simulink library "PowerFlowLib"  (R2016a)
settings: Solver=ode45  StartTime=0.0  StopTime=10.0  RelTol=1e-3
undefined symbols (not defined in the file or in its folder): Air, AirProp, C, F1, F2, Fanmap, Fld1, Fld2, Fluid, fueltankdata, HydProp, HydraulicLoad, IBFD_exc, L, LoadFluidProps, magnitude, MSSN, n_alghts, PumpProp, pwr_alghts, R_fd_exc, Rcore, Ts, VBFD_exc
libraries: PowerFlowLib x35, simulink x19, powerlib_extras x2, dspstat3 x2
(part 9 of 12)

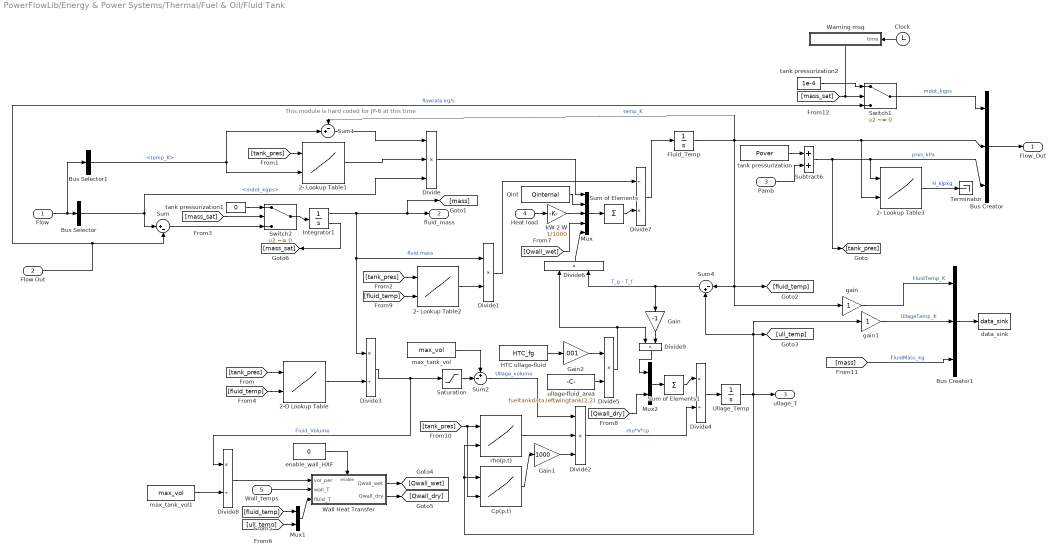
== system PowerFlowLib/Energy & Power Systems/Thermal/Fuel & Oil/Fluid Tank ==
  note: This module is hard coded for JP-8 at this time
  Flow : Inport
  Flow Out : Inport  Port=2
  Pamb : Inport  Port=3
  Heat load : Inport  Port=4
  Wall_temps : Inport  Port=5
  2- Lookup Table1 : Lookup_n-D  BreakpointsForDimension1=F1.P  BreakpointsForDimension2=F1.T  Table=F1.Cp_pt  RndMeth=Simplest  InputSameDT=on
  2- Lookup Table2 : Lookup_n-D  BreakpointsForDimension1=F1.P  BreakpointsForDimension2=F1.T  Table=F1.Cp_pt  RndMeth=Simplest  InputSameDT=on
  2- Lookup Table3 : Lookup_n-D  BreakpointsForDimension1=F1.P  BreakpointsForDimension2=F1.T  Table=F1.H_pt  RndMeth=Simplest  InputSameDT=on
  2-D Lookup Table : Lookup_n-D  BreakpointsForDimension1=F1.P  BreakpointsForDimension2=F1.T  Table=F1.Rho_pt  RndMeth=Simplest  InputSameDT=on
  Bus Creator : BusCreator  Inputs=3
  Bus Creator1 : BusCreator  Inputs=3
  Bus Selector : BusSelector  OutputSignals=mdot_kgps
  Bus Selector1 : BusSelector  OutputSignals=temp_K
  Clock : Clock
  Cp(p,t) : Lookup_n-D  BreakpointsForDimension1=AirProp.P  BreakpointsForDimension2=AirProp.T  Table=AirProp.Cp_pt  RndMeth=Simplest  InputSameDT=on
  Divide : Product  Inputs=***
  Divide{1,5..6,9} (4 alike) : Product  Inputs=**
  Divide2 : Product  Inputs=***
  Divide3 : Product  Inputs=*/
  Divide4 : Product  Inputs=*/
  Divide7 : Product  Inputs=/*
  Divide8 : Product  Inputs=*/
  Fluid_Temp : Integrator  InitialCondition=fld_Tint + 273.15  LimitOutput=on  UpperSaturationLimit=800  LowerSaturationLimit=eps
  Gain : Gain  Gain=-1
  Gain1 : Gain  Gain=1000
  Gain2 : Gain  Gain=.001
  HTC ullage-fluid : Constant  Value=HTC_fg
  Integrator1 : Integrator  InitialCondition=m_init  LimitOutput=on  LowerSaturationLimit=1  ShowSaturationPort=on
  Mux : Mux  Inputs=5
  Mux1 : Mux  Inputs=2
  Mux2 : Mux  Inputs=2
  Qint : Constant  Value=Qinternal
  Saturation : Saturate  UpperLimit=inf  LowerLimit=eps  ZeroCross=off
  Subtract6 : Sum
  Sum : Sum  Inputs=|+-
  Sum of Elements : Sum  Inputs=+
  Sum of Elements1 : Sum  Inputs=+
  Sum1 : Sum  Inputs=-+|
  Sum2 : Sum  Inputs=+-|
  Sum4 : Sum  Inputs=|-+
  Switch1 : Switch  Criteria=u2 ~= 0  Threshold=-1
  Switch2 : Switch  Criteria=u2 ~= 0  Threshold=-1
  Terminator : Terminator
  Ullage_Temp : Integrator  InitialCondition=ull_Tint + 273.15  LimitOutput=on  LowerSaturationLimit=eps
  Wall Heat Transfer : Subsystem  TreatAsAtomicUnit=on
  Warning msg : Subsystem  TreatAsAtomicUnit=on
  data_sink : PowerFlowLib/Support Functions//Tools/data_sink
  enable_wall_HXF : Constant  Value=0
  gain : Gain
  gain1 : Gain
  kW 2 W : Gain  Gain=1/1000
  max_tank_vol : Constant  Value=max_vol
  max_tank_vol1 : Constant  Value=max_vol
  rho(p,t) : Lookup_n-D  BreakpointsForDimension1=AirProp.P  BreakpointsForDimension2=AirProp.T  Table=AirProp.Rho_pt  RndMeth=Simplest  InputSameDT=on
  tank pressurization : Constant  Value=Pover
  tank pressurization1 : Constant  Value=0
  tank pressurization2 : Constant  Value=1e-4
  ullage-fluid_area : Constant  Value=fueltankdata.leftwingtank(2,2)
  Flow_Out : Outport
  fluid_mass : Outport  Port=2
  ullage_T : Outport  Port=3
  wires:
  [tank_pres] -> Cp(p,t)/2, rho(p,t)/1
  Gain2/1 -> Divide5/1
  enable_wall_HXF/1 -> Wall Heat Transfer/Enable
  [fluid_temp] -> 2- Lookup Table2/2
  [Qwall_wet] -> Mux/4
  [Qwall_dry] -> Mux2/2
  Divide9/1 -> Mux2/1
  Gain/1 -> Divide9/2
  Sum of Elements1/1 -> Divide4/1
  Mux2/1 -> Sum of Elements1/1
  Divide2/1 -> Divide4/2  "rho*V*cp"
  Divide6/1 -> Mux/5
  Wall Heat Transfer/2(Qwall_dry) -> [Qwall_dry]
  Wall Heat Transfer/1(Qwall_wet) -> [Qwall_wet]
  Mux1/1 -> Wall Heat Transfer/3(fluid_T)
  [ull_temp] -> Mux1/2
  [fluid_temp] -> Mux1/1
  Wall_temps/1 -> Wall Heat Transfer/2(wall_T)
  Divide8/1 -> Wall Heat Transfer/1(vol_per)
  [fluid_temp] -> 2-D Lookup Table/2
  Mux/1 -> Sum of Elements/1
  Sum of Elements/1 -> Divide7/2
  Heat load/1 -> kW 2 W/1
  Qint/1 -> Mux/2
  Divide/1 -> Mux/1
  Switch1/1 -> Bus Creator/1  "mdot_kgps"
  max_tank_vol1/1 -> Divide8/2
  [tank_pres] -> 2- Lookup Table2/1
  2- Lookup Table1/1 -> Divide/2
  [tank_pres] -> 2- Lookup Table1/1
  2-D Lookup Table/1 -> Divide3/2
  [tank_pres] -> 2-D Lookup Table/1
  Saturation/1 -> Sum2/2
  Bus Creator/1 -> Flow_Out/1
  Subtract6/1 -> [tank_pres], Bus Creator/3, 2- Lookup Table3/1  "pres_kPa"
  tank pressurization/1 -> Subtract6/1
  Pamb/1 -> Subtract6/2
  Divide5/1 -> Divide9/1, Divide6/1
  Divide7/1 -> Fluid_Temp/1
  Divide1/1 -> Divide7/1
  Sum4/1 -> Gain/1, Divide6/2  "T_g - T_f"
  ullage-fluid_area/1 -> Divide5/2
  HTC ullage-fluid/1 -> Gain2/1
  Fluid_Temp/1 -> [fluid_temp], Sum4/1, gain/1, Sum1/1, Bus Creator/2, 2- Lookup Table3/2  "temp_K"
  Ullage_Temp/1 -> Cp(p,t)/1, rho(p,t)/2, [ull_temp], Sum4/2, gain1/1, ullage_T/1
  Divide4/1 -> Ullage_Temp/1
  Sum2/1 -> Divide2/1  "Ullage_volume"
  max_tank_vol/1 -> Sum2/1
  Divide3/1 -> Divide8/1, Saturation/1  "Fluid_Volume"
  Cp(p,t)/1 -> Gain1/1
  rho(p,t)/1 -> Divide2/2
  2- Lookup Table2/1 -> Divide1/2
  Sum1/1 -> Divide/1
  Bus Selector1/1 -> 2- Lookup Table1/2, Sum1/2  "<temp_K>"
  Integrator1/1 -> Divide1/1, Divide3/1, [mass], fluid_mass/1  "fluid mass"
  Flow Out/1 -> Switch1/3, Sum/2  "flowrate kg/s"
  Bus Selector/1 -> Sum/1, Divide/3  "<mdot_kgps>"
  Flow/1 -> Bus Selector1/1, Bus Selector/1
  2- Lookup Table3/1 -> Terminator/1  "H_kJpkg"
  kW 2 W/1 -> Mux/3
  Bus Creator1/1 -> data_sink/1
  gain/1 -> Bus Creator1/1  "FluidTemp_K"
  gain1/1 -> Bus Creator1/2  "UllageTemp_K"
  [mass] -> Bus Creator1/3  "FluidMass_kg"
  [mass_sat] -> Switch1/2, Warning msg/Trigger
  tank pressurization2/1 -> Switch1/1
  Sum/1 -> Switch2/3
  Integrator1/2 -> [mass_sat]
  [mass_sat] -> Switch2/2
  tank pressurization1/1 -> Switch2/1
  Switch2/1 -> Integrator1/1
  Gain1/1 -> Divide2/3
  Clock/1 -> Warning msg/1(time)

== system PowerFlowLib/Energy & Power Systems/Thermal/Fuel & Oil/Fuel Control ==
  FuelNeed : Inport
  FuelFromPump : Inport  Port=2
  Bus Creator : BusCreator  Inputs=3
  Bus Creator1 : BusCreator  Inputs=3
  Bus Selector : BusSelector  OutputSignals=mdot_kgps,temp_K,pres_kPa
  Gain : Gain
  Gain1 : Gain
  Saturation : Saturate  UpperLimit=inf  LowerLimit=0
  Sum : Sum  Inputs=|+-
  Switch : Switch  Criteria=u2 > Threshold
  Fuel2Engine : Outport
  Fuel2Tank : Outport  Port=2
  wires:
  FuelFromPump/1 -> Bus Selector/1
  Bus Selector/1 -> Sum/1, Switch/3  "<mdot_kgps>"
  FuelNeed/1 -> Sum/2, Switch/1
  Sum/1 -> Saturation/1, Switch/2
  Bus Creator/1 -> Fuel2Tank/1
  Bus Selector/2 -> Bus Creator/2, Gain1/1  "<temp_K>"
  Saturation/1 -> Bus Creator/1  "mdot_kgps"
  Switch/1 -> Bus Creator1/1  "mdot_kgps"
  Bus Selector/3 -> Bus Creator/3, Gain/1  "<pres_kPa>"
  Bus Creator1/1 -> Fuel2Engine/1
  Gain/1 -> Bus Creator1/3  "pres_kPa"
  Gain1/1 -> Bus Creator1/2  "temp_K"

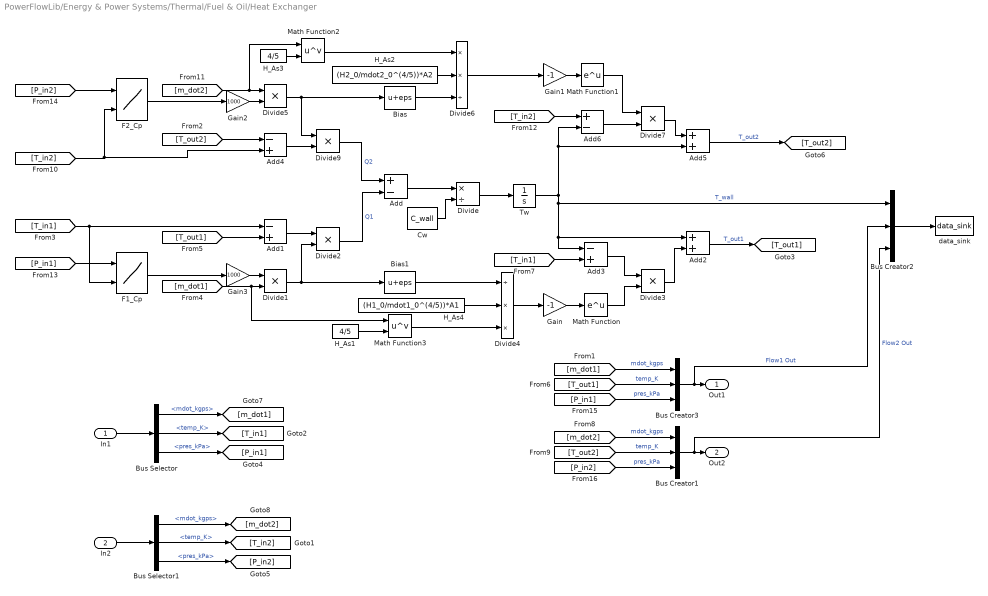
== system PowerFlowLib/Energy & Power Systems/Thermal/Fuel & Oil/Heat Exchanger ==
  In1 : Inport
  In2 : Inport  Port=2
  Add : Sum  Inputs=+-
  Add1 : Sum  Inputs=-+
  Add2 : Sum
  Add3 : Sum  Inputs=-+
  Add4 : Sum  Inputs=-+
  Add5 : Sum
  Add6 : Sum  Inputs=+-
  Bias : Bias  Bias=eps
  Bias1 : Bias  Bias=eps
  Bus Creator1 : BusCreator  Inputs=3
  Bus Creator2 : BusCreator  Inputs=3
  Bus Creator3 : BusCreator  Inputs=3
  Bus Selector : BusSelector  OutputSignals=mdot_kgps,temp_K,pres_kPa
  Bus Selector1 : BusSelector  OutputSignals=mdot_kgps,temp_K,pres_kPa
  Cw : Constant  Value=C_wall
  Divide : Product  Inputs=*/
  Divide{1..3,5,7,9} (6 alike) : Product  Inputs=**
  Divide4 : Product  Inputs=/**
  Divide6 : Product  Inputs=**/
  F1_Cp : Lookup_n-D  BreakpointsForDimension1=Fld1.P  BreakpointsForDimension2=Fld1.T  Table=Fld1.Cp_pt  ExtrapMethod=Clip  UseLastTableValue=on  RndMeth=Simplest  InputSameDT=on
  F2_Cp : Lookup_n-D  BreakpointsForDimension1=Fld2.P  BreakpointsForDimension2=Fld2.T  Table=Fld2.Cp_pt  ExtrapMethod=Clip  UseLastTableValue=on  RndMeth=Simplest  InputSameDT=on
  Gain : Gain  Gain=-1
  Gain1 : Gain  Gain=-1
  Gain2 : Gain  Gain=1000
  Gain3 : Gain  Gain=1000
  H_As1 : Constant  Value=4/5
  H_As2 : Constant  Value=(H2_0/mdot2_0^(4/5))*A2
  H_As3 : Constant  Value=4/5
  H_As4 : Constant  Value=(H1_0/mdot1_0^(4/5))*A1
  Math Function : Math  SaturateOnIntegerOverflow=on
  Math Function1 : Math  SaturateOnIntegerOverflow=on
  Math Function2 : Math  Operator=pow  SaturateOnIntegerOverflow=on
  Math Function3 : Math  Operator=pow  SaturateOnIntegerOverflow=on
  Tw : Integrator  InitialCondition=Tw_init + 273.15
  data_sink : PowerFlowLib/Support Functions//Tools/data_sink
  Out1 : Outport
  Out2 : Outport  Port=2
  wires:
  Divide/1 -> Tw/1
  Bias1/1 -> Divide4/1
  Bias/1 -> Divide6/3
  Bus Selector/1 -> [m_dot1]  "<mdot_kgps>"
  [T_in2] -> Add6/1
  Add6/1 -> Divide7/2
  Divide7/1 -> Add5/1
  Add5/1 -> [T_out2]  "T_out2"
  Math Function1/1 -> Divide7/1
  Gain1/1 -> Math Function1/1
  Divide6/1 -> Gain1/1
  H_As2/1 -> Divide6/2
  [m_dot2] -> Math Function2/1, Divide5/1
  F2_Cp/1 -> Gain2/1
  Divide5/1 -> Divide9/1, Bias/1
  [T_out2] -> Add4/1
  [T_in2] -> F2_Cp/2, Add4/2
  Add4/1 -> Divide9/2
  [m_dot2] -> Bus Creator1/1  "mdot_kgps"
  Bus Creator1/1 -> Bus Creator2/3, Out2/1  "Flow2 Out"
  Bus Selector1/2 -> [T_in2]  "<temp_K>"
  In2/1 -> Bus Selector1/1
  Gain/1 -> Math Function/1
  H_As4/1 -> Divide4/2
  Divide4/1 -> Gain/1
  Divide1/1 -> Bias1/1, Divide2/2
  Add1/1 -> Divide2/1
  Math Function/1 -> Divide3/2
  [T_in1] -> Add3/2
  [T_out1] -> Add1/2
  [m_dot1] -> Math Function3/1, Divide1/2
  [T_in1] -> F1_Cp/2, Add1/1
  Bus Selector/2 -> [T_in1]  "<temp_K>"
  Divide9/1 -> Add/1  "Q2"
  [m_dot1] -> Bus Creator3/1  "mdot_kgps"
  Bus Creator3/1 -> Bus Creator2/2, Out1/1  "Flow1 Out"
  Add3/1 -> Divide3/1
  Divide3/1 -> Add2/2
  Tw/1 -> Bus Creator2/1, Add3/1, Add2/1, Add5/2, Add6/2  "T_wall"
  Divide2/1 -> Add/2  "Q1"
  Add2/1 -> [T_out1]  "T_out1"
  F1_Cp/1 -> Gain3/1
  In1/1 -> Bus Selector/1
  Add/1 -> Divide/1
  Cw/1 -> Divide/2
  Math Function2/1 -> Divide6/1
  H_As3/1 -> Math Function2/2
  Math Function3/1 -> Divide4/3
  H_As1/1 -> Math Function3/2
  Bus Creator2/1 -> data_sink/1
  Bus Selector1/1 -> [m_dot2]  "<mdot_kgps>"
  Bus Selector/3 -> [P_in1]  "<pres_kPa>"
  Bus Selector1/3 -> [P_in2]  "<pres_kPa>"
  [P_in2] -> F2_Cp/1
  [P_in1] -> F1_Cp/1
  Gain2/1 -> Divide5/2
  Gain3/1 -> Divide1/1
  [T_out1] -> Bus Creator3/2  "temp_K"
  [T_out2] -> Bus Creator1/2  "temp_K"
  [P_in1] -> Bus Creator3/3  "pres_kPa"
  [P_in2] -> Bus Creator1/3  "pres_kPa"

== system PowerFlowLib/Energy & Power Systems/Thermal/Fuel & Oil/Stochastic Heat Loads ==
  Flow In : Inport
  Band-Limited White Noise : simulink/Sources/Band-Limited White Noise  Cov=noise_pwr  Ts=samp_time  seed=seed
  Bus Creator : BusCreator  Inputs=3
  Bus Selector : BusSelector  OutputSignals=temp_K,mdot_kgps,pres_kPa
  Gain : Gain
  Integrator : Integrator  LimitOutput=on  LowerSaturationLimit=0
  Sum : Sum  Inputs=++|
  Flow Out : Outport
  wires:
  Integrator/1 -> Sum/1
  Gain/1 -> Bus Creator/3  "pres_kPa"
  Bus Selector/3 -> Gain/1  "<pres_kPa>"
  Bus Selector/2 -> Bus Creator/2  "<mdot_kgps>"
  Sum/1 -> Bus Creator/1  "temp_K"
  Bus Creator/1 -> Flow Out/1
  Band-Limited White Noise/1 -> Integrator/1
  Bus Selector/1 -> Sum/2  "<temp_K>"
  Flow In/1 -> Bus Selector/1

== system PowerFlowLib/Energy & Power Systems/Electrical/Battery/BATTERY/BUS VOLTAGE ==
  VOLT/CELL : Inport
  NO_CELLS : Inport  Port=2
  PLOSS/CELL : Inport  Port=3
  Gain : Gain  Gain=NO_MODULES
  Product : Product  RndMeth=Zero
  Product1 : Product  RndMeth=Zero
  BUS VOLTAGE : Outport
  BATTERY_ PLOSS : Outport  Port=2
  wires:
  Gain/1 -> BATTERY_ PLOSS/1
  Product1/1 -> Gain/1
  PLOSS/CELL/1 -> Product1/1
  Product/1 -> BUS VOLTAGE/1
  NO_CELLS/1 -> Product1/2, Product/2
  VOLT/CELL/1 -> Product/1

== system PowerFlowLib/Energy & Power Systems/Electrical/Battery/BATTERY/NET  CHARGE//DISCHARGE DETECTION ==
  CT OUT : Inport
  CT IN : Inport  Port=2
  NO_MODULES : Inport  Port=3
  Add : Sum  Inputs=+++
  CHARGE : Product  RndMeth=Zero
  Compare To Zero : simulink/Logic and Bit Operations/Compare To Zero  relop=>  OutDataTypeStr=uint8
  Compare To Zero1 : simulink/Logic and Bit Operations/Compare To Zero  relop=<  OutDataTypeStr=uint8
  Compare To Zero2 : simulink/Logic and Bit Operations/Compare To Zero  relop===  OutDataTypeStr=uint8
  Constant : Constant
  Constant4 : Constant  Value=2
  Constant5 : Constant  Value=3
  DISCHARGE : Product  RndMeth=Zero
  DISCHARGE1 : Product  Inputs=*/  RndMeth=Zero
  DISCHARGE2 : Product  Inputs=*/  RndMeth=Zero
  OPEN CIRCUIT : Product  RndMeth=Zero
  Sum : Sum  Inputs=|+-
  CHG/DCHG SIGNAL : Outport
  DCHG CURRENT : Outport  Port=2
  CHG CURRENT : Outport  Port=3
  wires:
  DISCHARGE2/1 -> CHG CURRENT/1
  DISCHARGE1/1 -> DCHG CURRENT/1
  NO_MODULES/1 -> DISCHARGE2/2, DISCHARGE1/2
  Add/1 -> CHG/DCHG SIGNAL/1
  CT IN/1 -> DISCHARGE2/1, Sum/2
  CT OUT/1 -> DISCHARGE1/1, Sum/1
  Sum/1 -> Compare To Zero/1, Compare To Zero1/1, Compare To Zero2/1
  OPEN CIRCUIT/1 -> Add/3
  CHARGE/1 -> Add/2
  DISCHARGE/1 -> Add/1
  Constant5/1 -> OPEN CIRCUIT/2
  Compare To Zero2/1 -> OPEN CIRCUIT/1
  Constant4/1 -> CHARGE/2
  Compare To Zero1/1 -> CHARGE/1
  Constant/1 -> DISCHARGE/2
  Compare To Zero/1 -> DISCHARGE/1

== system PowerFlowLib/Energy & Power Systems/Electrical/Battery/BATTERY/SINGLE CELL VOLT OUT ==
  CHG_DCHG_SIGNAL : Inport
  DCHG CT : Inport  Port=2
  CHG CT : Inport  Port=3
  SOC : Inport  Port=4
  Add1 : Sum  Inputs=+-
  CHARGE : Subsystem
  Constant : Constant  Value=0
  DISCHARGE : Subsystem
  Demux : Demux  Outputs=2
  Memory : Memory  X0=3+13.433*INITIAL_SOC-90.038*INITIAL_SOC^2+284.33*INITIAL_SOC^3-453.64*INITIAL_SOC^4+355.88*INITIAL_SOC^5-108.97*INITIAL_SOC^6
  Multiport Switch : MultiPortSwitch  DiagnosticForDefault=None
  Mux : Mux  Inputs=2
  Mux1 : Mux  Inputs=2
  Mux2 : Mux  Inputs=2
  Saturation : Saturate  UpperLimit=inf  LowerLimit=0
  CELL VOLT : Outport
  POWER LOSS : Outport  Port=2
  wires:
  CHARGE/2(POWER LOSS) -> Mux/2
  Saturation/1 -> Mux1/1
  Memory/1 -> Mux2/1
  Constant/1 -> Mux2/2
  Demux/2 -> POWER LOSS/1
  Demux/1 -> CELL VOLT/1, Memory/1
  Multiport Switch/1 -> Demux/1
  Add1/1 -> CHARGE/1(NET BTRY CT), DISCHARGE/1(NET BTRY CT)
  SOC/1 -> CHARGE/2(SOC), DISCHARGE/2(SOC)
  CHG CT/1 -> Add1/2
  DCHG CT/1 -> Add1/1
  CHG_DCHG_SIGNAL/1 -> Multiport Switch/1
  Mux2/1 -> Multiport Switch/4
  Mux1/1 -> Multiport Switch/2
  Mux/1 -> Multiport Switch/3
  CHARGE/1(TERMINAL V) -> Mux/1
  DISCHARGE/2(POWER LOSS) -> Mux1/2
  DISCHARGE/1(TERMINAL V) -> Saturation/1

== system PowerFlowLib/Energy & Power Systems/Electrical/Battery/BATTERY/SOC  ==
  INITIAL SOC : Inport
  DCHG CT : Inport  Port=2
  CHG CT : Inport  Port=3
  CHG_DCHG_SIGNAL : Inport  Port=4
  Add1 : Sum  Inputs=+-
  Memory1 : Memory  X0=INITIAL_SOC
  Multiport Switch1 : MultiPortSwitch  DiagnosticForDefault=None
  SOC _ DISCHARGE : Subsystem
  SOC_CHARGE : Subsystem
  Saturation : Saturate  UpperLimit=1  LowerLimit=0
  DYNAMIC SOC : Outport
  NET DCHG CURRENT : Outport  Port=2
  wires:
  Saturation/1 -> Memory1/1, DYNAMIC SOC/1
  Memory1/1 -> Multiport Switch1/4
  Add1/1 -> SOC_CHARGE/2(NET BTRY CT), SOC _ DISCHARGE/2(NET BTRY CT), NET DCHG CURRENT/1
  INITIAL SOC/1 -> SOC_CHARGE/1(INITIAL SOC), SOC _ DISCHARGE/1(INTIAL SOC)
  Multiport Switch1/1 -> Saturation/1
  SOC_CHARGE/1(DYNAMIC SOC) -> Multiport Switch1/3
  DCHG CT/1 -> Add1/1
  CHG CT/1 -> Add1/2
  CHG_DCHG_SIGNAL/1 -> Multiport Switch1/1
  SOC _ DISCHARGE/1(DYNAMIC SOC) -> Multiport Switch1/2

== system PowerFlowLib/Energy & Power Systems/Electrical/Converters/Chopper (Averaged)/duty ratio ==
  d(t) : Inport
  Fcn : Fcn  Expr=1-u
  d1(t) : Outport
  d2(t) : Outport  Port=2
  wires:
  d(t)/1 -> d1(t)/1, Fcn/1
  Fcn/1 -> d2(t)/1

== system PowerFlowLib/Energy & Power Systems/Electrical/Inverters/ Inverter/Three-Phase Full Bridge Inverter CONSTANT FREQUENCY1 ==
  Vdc : Inport
  Inverter current : Inport  Port=2
  Add : Sum
  Constant : Constant  Value=Tr
  Constant1 : Constant  Value=Tf
  Constant2 : Constant  Value=Fsw
  Constant3 : Constant  Value=VCEsat
  No. of IGBT switches : Gain  Gain=Nsw
  "No. of series vol drops " : Gain  Gain=3
  Product : Product  RndMeth=Zero
  Switch Loss : Subsystem
  Total Loss : Outport
  Switching Loss : Outport  Port=2
  Conduction Loss : Outport  Port=3
  wires:
  Constant/1 -> Switch Loss/2(Trise)
  Constant1/1 -> Switch Loss/3(Tfall)
  Inverter current/1 -> Switch Loss/4(Inverter phase current), Product/1
  Switch Loss/1(Switch Loss) -> No. of IGBT switches/1
  Constant2/1 -> Switch Loss/5(Fsw mean)
  Vdc/1 -> Switch Loss/1(Vdc)
  Constant3/1 -> "No. of series vol drops "/1
  "No. of series vol drops "/1 -> Product/2
  Add/1 -> Total Loss/1
  No. of IGBT switches/1 -> Add/1, Switching Loss/1
  Product/1 -> Add/2, Conduction Loss/1

== system PowerFlowLib/Energy & Power Systems/Electrical/Inverters/1phs Inverter (2-level) - average/Dot Product ==
  In1 : Inport
  In2 : Inport  Port=2
  S-Function : S-Function  FunctionName=sdotproduct  SFunctionDeploymentMode=off  EnableBusSupport=off
  Out1 : Outport
  wires:
  S-Function/1 -> Out1/1
  In1/1 -> S-Function/1
  In2/1 -> S-Function/2

== system PowerFlowLib/Energy & Power Systems/Electrical/Inverters/1phs Inverter (2-level) - average/Dot Product1 ==
  In1 : Inport
  In2 : Inport  Port=2
  S-Function : S-Function  FunctionName=sdotproduct  SFunctionDeploymentMode=off  EnableBusSupport=off
  Out1 : Outport
  wires:
  S-Function/1 -> Out1/1
  In1/1 -> S-Function/1
  In2/1 -> S-Function/2

== system PowerFlowLib/Energy & Power Systems/Electrical/Inverters/1phs Inverter (2-level) - switching/2-level PWM ==
  d(t) : Inport
  Data Type Conversion : DataTypeConversion  SaturateOnIntegerOverflow=on  RndMeth=Zero
  Data Type Conversion1 : DataTypeConversion  SaturateOnIntegerOverflow=on  RndMeth=Zero
  Relational Operator : RelationalOperator  Operator=<=  InputSameDT=on
  Relational Operator1 : RelationalOperator  InputSameDT=on
  Tri(t) : Subsystem  mask(Repeating table){rep_seq_t=[0 1/f_s/2 1/f_s], rep_seq_y=[0 1 0]}
      mask prompts: rep_seq_t "Time values:"; rep_seq_y "Output values:"
      mask help: Output a repeating sequence of numbers specified in a table of time-value pairs. Values of time should be monotonically increasing.
      mask init:
      | if (length(rep_seq_t) ~= length(rep_seq_y)),
      |   error('Length of time vector and output vector must be the same.')
      | end
      | dbl_rep_seq_t = double(rep_seq_t);
      | dbl_rep_seq_y = double(rep_seq_y);
      | period = max(dbl_rep_seq_t) - min(dbl_rep_seq_t);
      | period = str2num(sprintf('%0.5g',period));
      | s = round(length(dbl_rep_seq_t)/50);
      | if s > 0
      |   pts = [1:s:length(dbl_rep_seq_t)];
      |   L   = length(pts);
      | else
      |   L   = length(dbl_rep_seq_t);
      |   pts = [1:L];
      | end
      | 
      | disp_seq_t = reshape(dbl_rep_seq_t(pts),L,1);
      | disp_seq_y = reshape(dbl_rep_seq_y(pts),L,1);
      | disp_period = max(disp_seq_t) - min(disp_seq_t);
      | 
      | disp_seq_t  = repmat(disp_seq_t,1,3) + (ones(L,1)*(disp_period*[0,1,2]));
      | disp_seq_t = [ disp_seq_t(:); disp_seq_t(end) ];
      | disp_seq_y = repmat(disp_seq_y,1,3);
      | disp_seq_y = [ disp_seq_y(:); disp_seq_y(1) ];
      mask Help: Repeats cycle given in table. Time values should be monotonically increasing.
      mask Display: plot( disp_seq_t, disp_seq_y )
  q1(t) : Outport
  q2(t) : Outport  Port=2
  wires:
  Relational Operator/1 -> Data Type Conversion/1
  Tri(t)/1(Out1) -> Relational Operator/1, Relational Operator1/1
  Relational Operator1/1 -> Data Type Conversion1/1
  d(t)/1 -> Relational Operator/2, Relational Operator1/2
  Data Type Conversion/1 -> q1(t)/1
  Data Type Conversion1/1 -> q2(t)/1

== system PowerFlowLib/Energy & Power Systems/Electrical/Inverters/1phs Inverter (2-level) - switching/Dot Product ==
  In1 : Inport
  In2 : Inport  Port=2
  S-Function : S-Function  FunctionName=sdotproduct  SFunctionDeploymentMode=off  EnableBusSupport=off
  Out1 : Outport
  wires:
  S-Function/1 -> Out1/1
  In1/1 -> S-Function/1
  In2/1 -> S-Function/2

== system PowerFlowLib/Energy & Power Systems/Electrical/Inverters/1phs Inverter (2-level) - switching/Dot Product1 ==
  In1 : Inport
  In2 : Inport  Port=2
  S-Function : S-Function  FunctionName=sdotproduct  SFunctionDeploymentMode=off  EnableBusSupport=off
  Out1 : Outport
  wires:
  S-Function/1 -> Out1/1
  In1/1 -> S-Function/1
  In2/1 -> S-Function/2

== system PowerFlowLib/Energy & Power Systems/Electrical/Inverters/Inverter (Average)/abc 2 dq ==
  I/P 3 phase : Inport
  angle : Inport  Port=2
  Constant : Constant  Value=2*pi/3
  Constant1 : Constant  Value=2*pi/3
  Demux2 : Demux  Outputs=3
  Gain1 : Gain  Gain=-2/3
  Gain2 : Gain  Gain=2/3
  Mux : Mux  Inputs=2
  Product{,1..5} (6 alike) : Product  RndMeth=Zero
  Sum : Sum  Inputs=|+-
  Sum1 : Sum  Inputs=|+++
  Sum2 : Sum  Inputs=|++
  Sum3 : Sum  Inputs=|+++
  Trigonometric Function : Trigonometry
  Trigonometric Function1 : Trigonometry  Operator=cos
  Trigonometric Function2 : Trigonometry
  Trigonometric Function3 : Trigonometry  Operator=cos
  Trigonometric Function4 : Trigonometry
  Trigonometric Function5 : Trigonometry  Operator=cos
  "O/P 2 phase " : Outport
  wires:
  angle/1 -> Trigonometric Function1/1, Trigonometric Function/1, Sum/1, Sum2/1
  I/P 3 phase/1 -> Demux2/1
  Mux/1 -> "O/P 2 phase "/1
  Trigonometric Function1/1 -> Product2/1
  Demux2/1 -> Product2/2, Product/2
  Constant/1 -> Sum/2
  Constant1/1 -> Sum2/2
  Sum/1 -> Trigonometric Function2/1, Trigonometric Function3/1
  Sum2/1 -> Trigonometric Function4/1, Trigonometric Function5/1
  Demux2/2 -> Product3/2, Product4/2
  Trigonometric Function3/1 -> Product3/1
  Trigonometric Function5/1 -> Product1/1
  Demux2/3 -> Product1/2, Product5/2
  Product2/1 -> Sum1/1
  Product3/1 -> Sum1/2
  Product1/1 -> Sum1/3
  Sum1/1 -> Gain2/1
  Gain2/1 -> Mux/1
  Trigonometric Function/1 -> Product/1
  Trigonometric Function2/1 -> Product4/1
  Trigonometric Function4/1 -> Product5/1
  Product/1 -> Sum3/1
  Product4/1 -> Sum3/2
  Product5/1 -> Sum3/3
  Sum3/1 -> Gain1/1
  Gain1/1 -> Mux/2

== system PowerFlowLib/Energy & Power Systems/Electrical/Loads/Constant Current Load/abc to qd0 ==
  note: abc to qd0 reference frame transform (using
      | Krause's notation q = direct axis, d = quadrature axis)
  V_a : Inport
  V_b : Inport  Port=2
  V_c : Inport  Port=3
  Fcn : Fcn  Expr=2/3*(u[1]*cos(0)+u[2]*cos(-2*pi/3)+u[3]*cos(2*pi/3))
  Fcn1 : Fcn  Expr=2/3*(u[1]*sin(0)+u[2]*sin(-2*pi/3)+u[3]*sin(2*pi/3))
  Fcn2 : Fcn  Expr=1/3*(u[1]+u[2]+u[3])
  Mux : Mux  Inputs=3
  V_q : Outport  InitialOutput=0
  V_d : Outport  Port=2  InitialOutput=0
  V_o : Outport  Port=3  InitialOutput=0
  wires:
  Fcn/1 -> V_q/1
  Fcn1/1 -> V_d/1
  Mux/1 -> Fcn/1, Fcn1/1, Fcn2/1
  V_c/1 -> Mux/3
  V_b/1 -> Mux/2
  V_a/1 -> Mux/1
  Fcn2/1 -> V_o/1

== system PowerFlowLib/Energy & Power Systems/Electrical/Loads/Constant Power Load/abc to qd0 ==
  note: abc to qd0 reference frame transform (using
      | Krause's notation q = direct axis, d = quadrature axis)
  V_a : Inport
  V_b : Inport  Port=2
  V_c : Inport  Port=3
  Fcn : Fcn  Expr=2/3*(u[1]*cos(0)+u[2]*cos(-2*pi/3)+u[3]*cos(2*pi/3))
  Fcn1 : Fcn  Expr=2/3*(u[1]*sin(0)+u[2]*sin(-2*pi/3)+u[3]*sin(2*pi/3))
  Fcn2 : Fcn  Expr=1/3*(u[1]+u[2]+u[3])
  Mux : Mux  Inputs=3
  V_q : Outport  InitialOutput=0
  V_d : Outport  Port=2  InitialOutput=0
  V_o : Outport  Port=3  InitialOutput=0
  wires:
  Fcn/1 -> V_q/1
  Fcn1/1 -> V_d/1
  Mux/1 -> Fcn/1, Fcn1/1, Fcn2/1
  V_c/1 -> Mux/3
  V_b/1 -> Mux/2
  V_a/1 -> Mux/1
  Fcn2/1 -> V_o/1

== system PowerFlowLib/Energy & Power Systems/Electrical/Loads/Enabled_AC_Loadloss/Enabled Subsystem ==
  "Vdq0 " : Inport
  CURRENT BASED LOADS : Subsystem
  IMPEDANCE BASED LOADS : Subsystem
  POWER BASED LOADS : Subsystem
  Sum of Elements : Sum  Inputs=+++
  Idq0 : Outport
  loss : Outport  Port=2
  wires:
  "Vdq0 "/1 -> IMPEDANCE BASED LOADS/1(Vdq0), POWER BASED LOADS/1(Vdq0)
  POWER BASED LOADS/1(Idq0) -> Sum of Elements/1
  CURRENT BASED LOADS/1(Idqo) -> Sum of Elements/2
  Sum of Elements/1 -> Idq0/1
  IMPEDANCE BASED LOADS/1(Idq0) -> Sum of Elements/3
  POWER BASED LOADS/2(loss) -> loss/1

== system PowerFlowLib/Energy & Power Systems/Electrical/Loads/Enabled_AC_Loadloss/Enabled Subsystem1 ==
  "Vdq0 " : Inport
  Ext vector : Inport  Port=2
  CURRENT BASED LOADS : Subsystem
  Demux : Demux  Outputs=3
  POWER BASED LOADS : Subsystem
  Sum of Elements : Sum
  Idq0 : Outport
  wires:
  CURRENT BASED LOADS/1(Idqo) -> Sum of Elements/2
  POWER BASED LOADS/1(Idq0) -> Sum of Elements/1
  Sum of Elements/1 -> Idq0/1
  Ext vector/1 -> Demux/1
  "Vdq0 "/1 -> POWER BASED LOADS/1(Vdq0)
  Demux/1 -> POWER BASED LOADS/2(P)
  Demux/2 -> POWER BASED LOADS/3(Q)
  Demux/3 -> CURRENT BASED LOADS/1(Iconst RMS)

== system PowerFlowLib/Energy & Power Systems/Electrical/Loss Estimation/Three-Phase ACTIVE RECTIFIER/Switch Loss ==
  Vdc : Inport
  Trise : Inport  Port=2
  Tfall : Inport  Port=3
  Inverter Phae current : Inport  Port=4
  Fsw mean : Inport  Port=5
  Add : Sum
  Divide : Product  Inputs=****
  Gain : Gain  Gain=0.5
  Switching Loss : Outport
  wires:
  Gain/1 -> Divide/2
  Vdc/1 -> Divide/1
  Trise/1 -> Add/1
  Tfall/1 -> Add/2
  Add/1 -> Gain/1
  Inverter Phae current/1 -> Divide/3
  Fsw mean/1 -> Divide/4
  Divide/1 -> Switching Loss/1

== system PowerFlowLib/Energy & Power Systems/Electrical/Loss Estimation/Three-Phase ACTIVE RECTIFIER/Switching Frequency ==
  Vdc : Inport
  Source Vol (RMS) : Inport  Port=2
  H-Band : Inport  Port=3
  Lls : Inport  Port=4
  theta : Inport  Port=5
  Add : Sum  Inputs=+-
  Divide : Product  Inputs=**
  Divide1 : Product  Inputs=*/
  Divide2 : Product  Inputs=***
  Gain : Gain  Gain=sqrt(2)
  Gain1 : Gain  Gain=1/(2*pi)
  Gain2 : Gain  Gain=4
  Math Function : Math  Operator=square  SaturateOnIntegerOverflow=on
  Math Function1 : Math  Operator=square  SaturateOnIntegerOverflow=on
  Mean : dspstat3/Mean  run=on  reset_popup=None  InputProcessing=Columns as channels (frame based)  directionMode=Each column  dimension=1  treatSBRowAsCol=on  roiEnable=off  roiType=Rectangles  roiPortion=Entire ROI  roiOutput=Individual statistics for each ROI  roiFlag=off  outputDataTypeStr=Inherit: Same as accumulator  outputLastDataTypeStr=Inherit: Same as accumulator  outputMin=[]  outputMax=[]  roundingMode=Floor  overflowMode=off
  Scope8 : Scope  NumInputPorts=4
  Sine : simulink/Lookup Tables/Sine  Formula=sin(2*pi*u)  NumDataPoints=(2^5)+1  OutputWordLength=16
  Zero-Order Hold : ZeroOrderHold  SampleTime=Ts
  Inst. fsw : Outport
  Mean fsw : Outport  Port=2
  wires:
  Vdc/1 -> Divide2/3, Math Function/1, Scope8/1
  Source Vol (RMS)/1 -> Gain/1
  theta/1 -> Gain1/1
  Gain/1 -> Divide/1
  Math Function/1 -> Add/1
  Divide/1 -> Math Function1/1
  Sine/1 -> Divide/2
  Gain1/1 -> Sine/1
  Math Function1/1 -> Add/2
  Add/1 -> Divide1/1, Scope8/2
  H-Band/1 -> Gain2/1
  Gain2/1 -> Divide2/1
  Lls/1 -> Divide2/2
  Divide2/1 -> Divide1/2, Scope8/4
  Divide1/1 -> Zero-Order Hold/1, Inst. fsw/1, Scope8/3
  Mean/1 -> Mean fsw/1
  Zero-Order Hold/1 -> Mean/1

== system PowerFlowLib/Energy & Power Systems/Electrical/Loss Estimation/Three-Phase Full Bridge Inverter CONSTANT FREQUENCY/Switch Loss ==
  Vdc : Inport
  Trise : Inport  Port=2
  Tfall : Inport  Port=3
  Inverter phase current : Inport  Port=4
  Fsw mean : Inport  Port=5
  Add : Sum
  Divide : Product  Inputs=****
  Gain : Gain  Gain=0.5
  Switch Loss : Outport
  wires:
  Vdc/1 -> Divide/1
  Trise/1 -> Add/1
  Tfall/1 -> Add/2
  Add/1 -> Gain/1
  Inverter phase current/1 -> Divide/3
  Fsw mean/1 -> Divide/4
  Divide/1 -> Switch Loss/1
  Gain/1 -> Divide/2

== system PowerFlowLib/Energy & Power Systems/Electrical/Loss Estimation/Three-Phase Full Bridge Inverter VARIABLE FREQUENCY/Switch Loss ==
  Vdc : Inport
  Trise : Inport  Port=2
  Tfall : Inport  Port=3
  Inverter Phae current : Inport  Port=4
  Fsw mean : Inport  Port=5
  Add : Sum
  Divide : Product  Inputs=****
  Gain : Gain  Gain=0.5
  Switching Loss : Outport
  wires:
  Divide/1 -> Switching Loss/1
  Fsw mean/1 -> Divide/4
  Inverter Phae current/1 -> Divide/3
  Add/1 -> Gain/1
  Tfall/1 -> Add/2
  Trise/1 -> Add/1
  Vdc/1 -> Divide/1
  Gain/1 -> Divide/2

== system PowerFlowLib/Energy & Power Systems/Electrical/Loss Estimation/Three-Phase Full Bridge Inverter VARIABLE FREQUENCY/Switching Frequency ==
  Vdc : Inport
  Machine vol (RMS) : Inport  Port=2
  H-Band : Inport  Port=3
  Lls : Inport  Port=4
  theta : Inport  Port=5
  Add : Sum  Inputs=+-
  Divide : Product  Inputs=**
  Divide1 : Product  Inputs=*/
  Divide2 : Product  Inputs=***
  Gain : Gain  Gain=sqrt(2)
  Gain1 : Gain  Gain=1/(2*pi)
  Gain2 : Gain  Gain=4
  Math Function : Math  Operator=square  SaturateOnIntegerOverflow=on
  Math Function1 : Math  Operator=square  SaturateOnIntegerOverflow=on
  Mean : dspstat3/Mean  run=on  reset_popup=None  InputProcessing=Columns as channels (frame based)  directionMode=Each column  dimension=1  treatSBRowAsCol=on  roiEnable=off  roiType=Rectangles  roiPortion=Entire ROI  roiOutput=Individual statistics for each ROI  roiFlag=off  outputDataTypeStr=Inherit: Same as accumulator  outputLastDataTypeStr=Inherit: Same as accumulator  outputMin=[]  outputMax=[]  roundingMode=Floor  overflowMode=off
  Scope8 : Scope  NumInputPorts=4
  Sine : simulink/Lookup Tables/Sine  Formula=sin(2*pi*u)  NumDataPoints=(2^5)+1  OutputWordLength=16
  Zero-Order Hold : ZeroOrderHold  SampleTime=Ts
  Inst. fsw : Outport
  Mean fsw : Outport  Port=2
  wires:
  Zero-Order Hold/1 -> Mean/1
  Mean/1 -> Mean fsw/1
  Divide1/1 -> Scope8/3, Inst. fsw/1, Zero-Order Hold/1
  Divide2/1 -> Scope8/4, Divide1/2
  Lls/1 -> Divide2/2
  Gain2/1 -> Divide2/1
  H-Band/1 -> Gain2/1
  Add/1 -> Scope8/2, Divide1/1
  Math Function1/1 -> Add/2
  Gain1/1 -> Sine/1
  Sine/1 -> Divide/2
  Divide/1 -> Math Function1/1
  Math Function/1 -> Add/1
  Gain/1 -> Divide/1
  theta/1 -> Gain1/1
  Machine vol (RMS)/1 -> Gain/1
  Vdc/1 -> Scope8/1, Math Function/1, Divide2/3

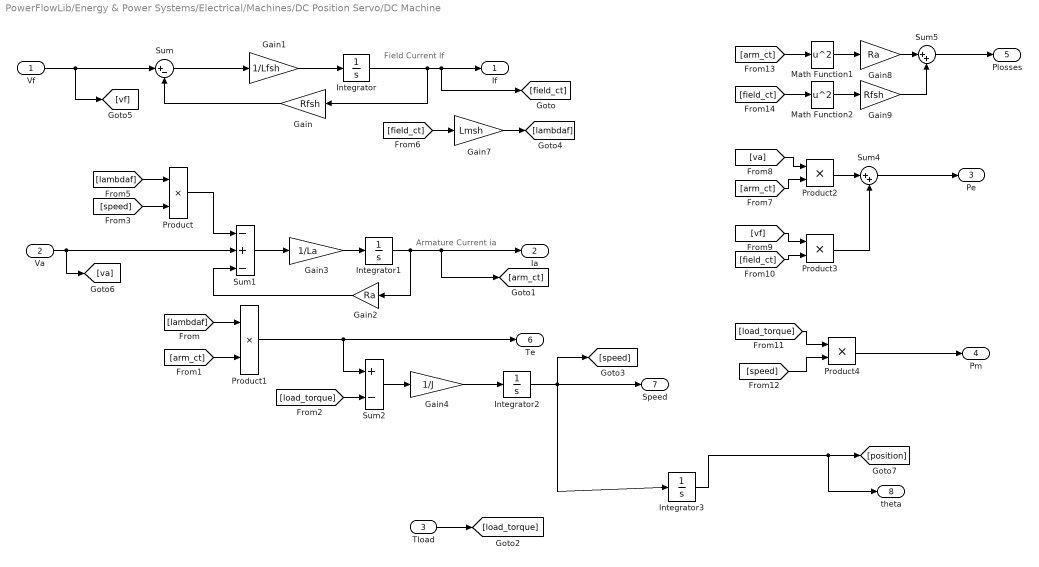
== system PowerFlowLib/Energy & Power Systems/Electrical/Machines/DC Position Servo/DC Machine ==
  note: Armature Current ia
  note: Field Current If
  Vf : Inport
  Va : Inport  Port=2
  Tload : Inport  Port=3
  Gain : Gain  Gain=Rfsh
  Gain1 : Gain  Gain=1/Lfsh
  Gain2 : Gain  Gain=Ra
  Gain3 : Gain  Gain=1/La
  Gain4 : Gain  Gain=1/J
  Gain7 : Gain  Gain=Lmsh
  Gain8 : Gain  Gain=Ra
  Gain9 : Gain  Gain=Rfsh
  Integrator : Integrator
  Integrator1 : Integrator
  Integrator2 : Integrator
  Integrator3 : Integrator  ZeroCross=off
  Math Function1 : Math  Operator=square  SaturateOnIntegerOverflow=on
  Math Function2 : Math  Operator=square  SaturateOnIntegerOverflow=on
  Product{,1..4} (5 alike) : Product  RndMeth=Zero
  Sum : Sum  Inputs=|+-
  Sum1 : Sum  Inputs=-+-
  Sum2 : Sum  Inputs=+-
  Sum4 : Sum  Inputs=|++
  Sum5 : Sum  Inputs=|++
  If : Outport
  Ia : Outport  Port=2
  Pe : Outport  Port=3
  Pm : Outport  Port=4
  Plosses : Outport  Port=5
  Te : Outport  Port=6
  Speed : Outport  Port=7
  theta : Outport  Port=8
  wires:
  Gain/1 -> Sum/2
  Sum/1 -> Gain1/1
  Integrator/1 -> [field_ct], If/1, Gain/1
  Sum1/1 -> Gain3/1
  Gain3/1 -> Integrator1/1
  Integrator1/1 -> Gain2/1, [arm_ct], Ia/1
  Product1/1 -> Sum2/1, Te/1
  Sum2/1 -> Gain4/1
  Gain4/1 -> Integrator2/1
  Gain1/1 -> Integrator/1
  Product/1 -> Sum1/1
  Gain2/1 -> Sum1/3
  [lambdaf] -> Product1/1
  [arm_ct] -> Product1/2
  [load_torque] -> Sum2/2
  [speed] -> Product/2
  [lambdaf] -> Product/1
  [field_ct] -> Gain7/1
  Gain7/1 -> [lambdaf]
  Vf/1 -> Sum/1, [vf]
  Va/1 -> Sum1/2, [va]
  [va] -> Product2/1
  [arm_ct] -> Product2/2
  Product2/1 -> Sum4/1
  [vf] -> Product3/1
  [field_ct] -> Product3/2
  Product3/1 -> Sum4/2
  Sum4/1 -> Pe/1
  [load_torque] -> Product4/1
  [speed] -> Product4/2
  Product4/1 -> Pm/1
  Integrator3/1 -> [position], theta/1
  [arm_ct] -> Math Function1/1
  Math Function1/1 -> Gain8/1
  Gain8/1 -> Sum5/1
  [field_ct] -> Math Function2/1
  Math Function2/1 -> Gain9/1
  Gain9/1 -> Sum5/2
  Sum5/1 -> Plosses/1
  Integrator2/1 -> Speed/1, [speed], Integrator3/1
  Tload/1 -> [load_torque]

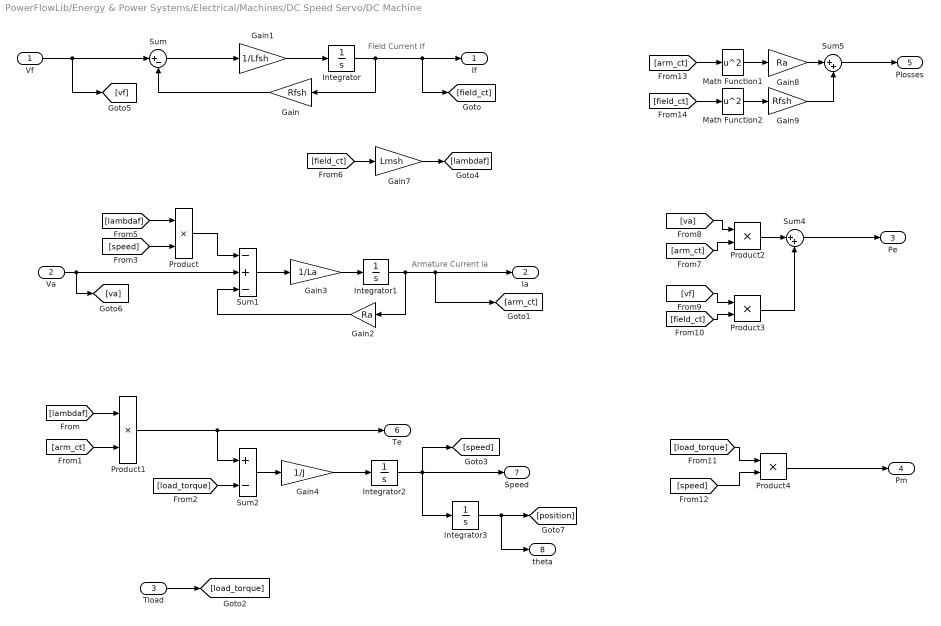
== system PowerFlowLib/Energy & Power Systems/Electrical/Machines/DC Speed Servo/DC Machine ==
  note: Field Current If
  note: Armature Current ia
  Vf : Inport
  Va : Inport  Port=2
  Tload : Inport  Port=3
  Gain : Gain  Gain=Rfsh
  Gain1 : Gain  Gain=1/Lfsh
  Gain2 : Gain  Gain=Ra
  Gain3 : Gain  Gain=1/La
  Gain4 : Gain  Gain=1/J
  Gain7 : Gain  Gain=Lmsh
  Gain8 : Gain  Gain=Ra
  Gain9 : Gain  Gain=Rfsh
  Integrator : Integrator
  Integrator1 : Integrator
  Integrator2 : Integrator
  Integrator3 : Integrator  ZeroCross=off
  Math Function1 : Math  Operator=square  SaturateOnIntegerOverflow=on
  Math Function2 : Math  Operator=square  SaturateOnIntegerOverflow=on
  Product{,1..4} (5 alike) : Product  RndMeth=Zero
  Sum : Sum  Inputs=|+-
  Sum1 : Sum  Inputs=-+-
  Sum2 : Sum  Inputs=+-
  Sum4 : Sum  Inputs=|++
  Sum5 : Sum  Inputs=|++
  If : Outport
  Ia : Outport  Port=2
  Pe : Outport  Port=3
  Pm : Outport  Port=4
  Plosses : Outport  Port=5
  Te : Outport  Port=6
  Speed : Outport  Port=7
  theta : Outport  Port=8
  wires:
  Tload/1 -> [load_torque]
  Integrator2/1 -> Integrator3/1, [speed], Speed/1
  Sum5/1 -> Plosses/1
  Gain9/1 -> Sum5/2
  Math Function2/1 -> Gain9/1
  [field_ct] -> Math Function2/1
  Gain8/1 -> Sum5/1
  Math Function1/1 -> Gain8/1
  [arm_ct] -> Math Function1/1
  Product4/1 -> Pm/1
  [speed] -> Product4/2
  [load_torque] -> Product4/1
  Sum4/1 -> Pe/1
  Product3/1 -> Sum4/2
  [field_ct] -> Product3/2
  [vf] -> Product3/1
  Product2/1 -> Sum4/1
  [arm_ct] -> Product2/2
  [va] -> Product2/1
  Va/1 -> [va], Sum1/2
  Vf/1 -> [vf], Sum/1
  Gain7/1 -> [lambdaf]
  [field_ct] -> Gain7/1
  [lambdaf] -> Product/1
  [speed] -> Product/2
  [load_torque] -> Sum2/2
  [arm_ct] -> Product1/2
  [lambdaf] -> Product1/1
  Gain2/1 -> Sum1/3
  Product/1 -> Sum1/1
  Gain1/1 -> Integrator/1
  Gain4/1 -> Integrator2/1
  Sum2/1 -> Gain4/1
  Product1/1 -> Te/1, Sum2/1
  Integrator1/1 -> Ia/1, [arm_ct], Gain2/1
  Gain3/1 -> Integrator1/1
  Sum1/1 -> Gain3/1
  Integrator/1 -> If/1, [field_ct], Gain/1
  Sum/1 -> Gain1/1
  Gain/1 -> Sum/2
  Integrator3/1 -> [position], theta/1

== system PowerFlowLib/Energy & Power Systems/Electrical/Machines/Induction motor/D-axis block ==
  vds : Inport
  wr*pqr : Inport  Port=2
  Integrator : Integrator
  Integrator1 : Integrator
  Mux : Mux  Inputs=3
  Mux1 : Mux  Inputs=3
  Mux2 : Mux  Inputs=2
  Mux3 : Mux  Inputs=2
  i_ds : Fcn  Expr=1/IM_Xls*(u[2]-u[1])
  pmd : Fcn  Expr=IM_XM*(u[1]/IM_Xls+u[2]/IM_Xplr)
  psi_dr : Fcn  Expr=IM_wb*(-u[2]/IM_wb+IM_rrp/IM_Xplr*(u[1]-u[3]))
  psi_ds : Fcn  Expr=IM_wb*(u[2]+IM_rs/IM_Xls*(u[3]-u[1]))
  pds : Outport
  ids : Outport  Port=2
  pdr : Outport  Port=3
  wires:
  i_ds/1 -> ids/1
  Mux3/1 -> i_ds/1
  wr*pqr/1 -> Mux1/2
  Integrator1/1 -> pdr/1, Mux2/2, Mux1/3
  Integrator/1 -> pds/1, Mux3/2, Mux2/1, Mux/1
  psi_dr/1 -> Integrator1/1
  psi_ds/1 -> Integrator/1
  Mux2/1 -> pmd/1
  Mux1/1 -> psi_dr/1
  pmd/1 -> Mux1/1, Mux3/1, Mux/3
  Mux/1 -> psi_ds/1
  vds/1 -> Mux/2

== system PowerFlowLib/Energy & Power Systems/Electrical/Machines/Induction motor/Power Loss Measurement ==
  vqd0s : Inport
  iqd0s : Inport  Port=2
  T_em : Inport  Port=3
  wr_mech : Inport  Port=4
  Gain1 : Gain  Gain=1/Rcore
  Gain2 : Gain  Gain=[3/2 3/2 1]
  Gain3 : Gain  Gain=IM_rs
  Gain4 : Gain  Gain=[3/2 3/2 1].^2
  Gain5 : Gain  Gain=[3/2 3/2 1].^2
  Math Function : Math  Operator=square  SaturateOnIntegerOverflow=on
  Math Function1 : Math  Operator=square  SaturateOnIntegerOverflow=on
  Product : Product  RndMeth=Zero
  Product1 : Product  RndMeth=Zero
  Sum : Sum  Inputs=+
  Sum1 : Sum  Inputs=+-|
  Sum2 : Sum  Inputs=+
  Sum4 : Sum  Inputs=+
  Sum5 : Sum
  P_el : Outport
  P_m : Outport  Port=2
  P_loss : Outport  Port=3
  P_el_loss : Outport  Port=4
  wires:
  Product/1 -> Gain2/1
  vqd0s/1 -> Product/1, Math Function/1
  iqd0s/1 -> Product/2, Math Function1/1
  Gain2/1 -> Sum/1
  Sum/1 -> P_el/1, Sum1/1
  Product1/1 -> P_m/1, Sum1/2
  T_em/1 -> Product1/1
  wr_mech/1 -> Product1/2
  Sum1/1 -> P_loss/1
  Gain1/1 -> Gain5/1
  Gain3/1 -> Gain4/1
  Math Function/1 -> Gain1/1
  Math Function1/1 -> Gain3/1
  Sum2/1 -> Sum5/1
  Sum4/1 -> Sum5/2
  Sum5/1 -> P_el_loss/1
  Gain4/1 -> Sum4/1  "Copper Losses"
  Gain5/1 -> Sum2/1  "Core Loss"

== system PowerFlowLib/Energy & Power Systems/Electrical/Machines/Induction motor/Q-axis block ==
  vqs : Inport
  wr*pdr : Inport  Port=2
  Integrator : Integrator
  Integrator1 : Integrator
  Mux : Mux  Inputs=3
  Mux1 : Mux  Inputs=3
  Mux2 : Mux  Inputs=2
  Mux3 : Mux  Inputs=2
  i_qs : Fcn  Expr=1/IM_Xls*(u[2]-u[1])
  pmq : Fcn  Expr=IM_XM*(u[1]/IM_Xls+u[2]/IM_Xplr)
  psi_qr : Fcn  Expr=IM_wb*(u[2]/IM_wb+IM_rrp/IM_Xplr*(u[1]-u[3]))
  psi_qs : Fcn  Expr=IM_wb*(u[2]+IM_rs/IM_Xls*(u[3]-u[1]))
  pqs : Outport
  iqs : Outport  Port=2
  pqr : Outport  Port=3
  wires:
  i_qs/1 -> iqs/1
  Mux3/1 -> i_qs/1
  wr*pdr/1 -> Mux1/2
  Integrator1/1 -> pqr/1, Mux2/2, Mux1/3
  Integrator/1 -> pqs/1, Mux3/2, Mux2/1, Mux/1
  psi_qr/1 -> Integrator1/1
  psi_qs/1 -> Integrator/1
  Mux2/1 -> pmq/1
  Mux1/1 -> psi_qr/1
  pmq/1 -> Mux1/1, Mux3/1, Mux/3
  Mux/1 -> psi_qs/1
  vqs/1 -> Mux/2

== system PowerFlowLib/Energy & Power Systems/Electrical/Machines/Permanent Magnet Synchronous Generator1/Generator Power Loss1 ==
  Ploss : Inport
  Tamb : Inport  Port=2
  Gain1 : Gain  Gain=1/mc_exciter
  Heat Trasnfer : Subsystem
  Integrator : Integrator  InitialConditionSource=external
  Sum : Sum  Inputs=|+-
  Ts : Outport
  Pdiss : Outport  Port=2
  wires:
  Gain1/1 -> Integrator/1
  Heat Trasnfer/1(Pdiss) -> Pdiss/1, Sum/2
  Ploss/1 -> Sum/1
  Sum/1 -> Gain1/1
  Integrator/1 -> Heat Trasnfer/2(Ts), Ts/1
  Tamb/1 -> Heat Trasnfer/1(Tamb), Integrator/2

== system PowerFlowLib/Energy & Power Systems/Electrical/Machines/Permanent Magnet Synchronous Generator1/Power Loss Measurement ==
  vqd0s : Inport
  iqd0s : Inport  Port=2
  T_em : Inport  Port=3
  wr_mech : Inport  Port=4
  Gain1 : Gain  Gain=1e-10
  Gain2 : Gain  Gain=[3/2 3/2 1]
  Gain3 : Gain  Gain=Rs_pm
  Gain4 : Gain  Gain=[3/2 3/2 1].^2
  Gain5 : Gain  Gain=[3/2 3/2 1].^2
  Math Function : Math  Operator=square  SaturateOnIntegerOverflow=on
  Math Function1 : Math  Operator=square  SaturateOnIntegerOverflow=on
  Product : Product  RndMeth=Zero
  Product1 : Product  RndMeth=Zero
  Sum : Sum  Inputs=+
  Sum1 : Sum  Inputs=-+|
  Sum2 : Sum  Inputs=+
  Sum4 : Sum  Inputs=+
  Sum5 : Sum
  P_el : Outport
  P_m : Outport  Port=2
  P_loss : Outport  Port=3
  P_el_loss : Outport  Port=4
  wires:
  Product/1 -> Gain2/1
  vqd0s/1 -> Product/1, Math Function/1
  iqd0s/1 -> Product/2, Math Function1/1
  Gain2/1 -> Sum/1
  Sum/1 -> P_el/1, Sum1/1
  Product1/1 -> P_m/1, Sum1/2
  T_em/1 -> Product1/1
  wr_mech/1 -> Product1/2
  Sum1/1 -> P_loss/1
  Gain1/1 -> Gain5/1
  Gain3/1 -> Gain4/1
  Math Function/1 -> Gain1/1
  Math Function1/1 -> Gain3/1
  Sum2/1 -> Sum5/1
  Sum4/1 -> Sum5/2
  Sum5/1 -> P_el_loss/1
  Gain4/1 -> Sum4/1  "Copper Losses"
  Gain5/1 -> Sum2/1  "Core Loss"

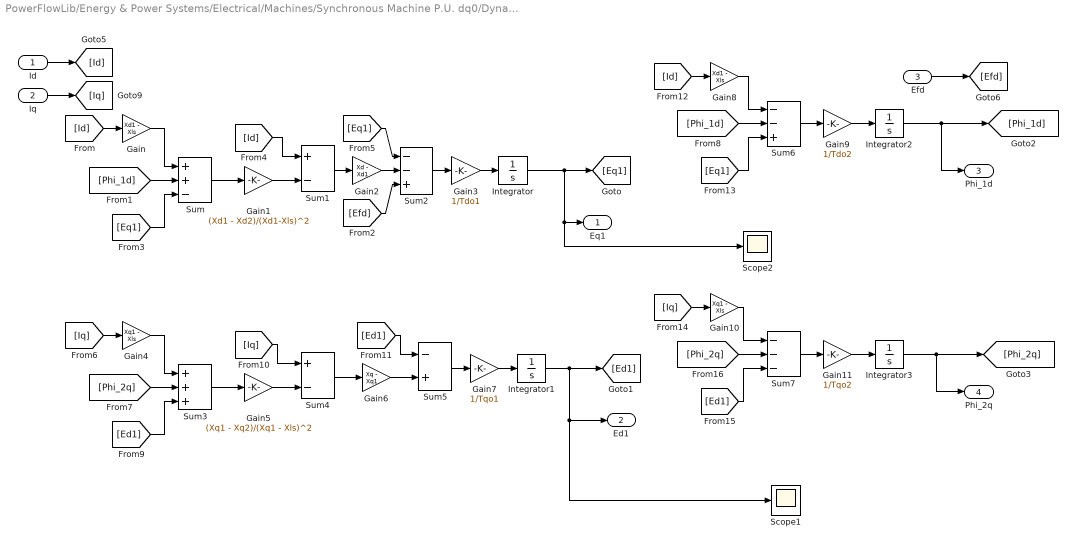
== system PowerFlowLib/Energy & Power Systems/Electrical/Machines/Synchronous Machine P.U. dq0/Dynamics ==
  Id : Inport
  Iq : Inport  Port=2
  Efd : Inport  Port=3
  Gain : Gain  Gain=Xd1 - Xls
  Gain1 : Gain  Gain=(Xd1 - Xd2)/(Xd1-Xls)^2
  Gain10 : Gain  Gain=Xq1 - Xls
  Gain11 : Gain  Gain=1/Tqo2
  Gain2 : Gain  Gain=Xd - Xd1
  Gain3 : Gain  Gain=1/Tdo1
  Gain4 : Gain  Gain=Xq1 - Xls
  Gain5 : Gain  Gain=(Xq1 - Xq2)/(Xq1 - Xls)^2
  Gain6 : Gain  Gain=Xq - Xq1
  Gain7 : Gain  Gain=1/Tqo1
  Gain8 : Gain  Gain=Xd1 - Xls
  Gain9 : Gain  Gain=1/Tdo2
  Integrator{,1..3} (4 alike) : Integrator
  Scope1 : Scope
  Scope2 : Scope
  Sum : Sum  Inputs=++-
  Sum1 : Sum  Inputs=+-
  Sum2 : Sum  Inputs=--+
  Sum3 : Sum  Inputs=+++
  Sum4 : Sum  Inputs=+-
  Sum5 : Sum  Inputs=-+
  Sum6 : Sum  Inputs=--+
  Sum7 : Sum  Inputs=---
  Eq1 : Outport
  Ed1 : Outport  Port=2
  Phi_1d : Outport  Port=3
  Phi_2q : Outport  Port=4
  wires:
  Efd/1 -> [Efd]
  Iq/1 -> [Iq]
  Id/1 -> [Id]
  Integrator3/1 -> Phi_2q/1, [Phi_2q]
  Gain11/1 -> Integrator3/1
  Sum7/1 -> Gain11/1
  [Ed1] -> Sum7/3
  [Phi_2q] -> Sum7/2
  Gain10/1 -> Sum7/1
  [Iq] -> Gain10/1
  Integrator2/1 -> Phi_1d/1, [Phi_1d]
  Gain9/1 -> Integrator2/1
  Sum6/1 -> Gain9/1
  [Eq1] -> Sum6/3
  [Phi_1d] -> Sum6/2
  Gain8/1 -> Sum6/1
  [Id] -> Gain8/1
  Gain7/1 -> Integrator1/1
  Sum5/1 -> Gain7/1
  Gain6/1 -> Sum5/2
  [Ed1] -> Sum5/1
  Sum4/1 -> Gain6/1
  Gain5/1 -> Sum4/2
  [Iq] -> Sum4/1
  Sum3/1 -> Gain5/1
  [Ed1] -> Sum3/3
  [Phi_2q] -> Sum3/2
  Gain4/1 -> Sum3/1
  [Iq] -> Gain4/1
  Integrator1/1 -> Scope1/1, Ed1/1, [Ed1]
  Gain3/1 -> Integrator/1
  Sum2/1 -> Gain3/1
  [Efd] -> Sum2/3
  Gain2/1 -> Sum2/2
  [Eq1] -> Sum2/1
  Sum1/1 -> Gain2/1
  Gain1/1 -> Sum1/2
  [Id] -> Sum1/1
  Sum/1 -> Gain1/1
  [Eq1] -> Sum/3
  [Phi_1d] -> Sum/2
  Gain/1 -> Sum/1
  [Id] -> Gain/1
  Integrator/1 -> Scope2/1, Eq1/1, [Eq1]

== system PowerFlowLib/Energy & Power Systems/Electrical/Machines/Synchronous Machine P.U. dq0/Electromagnetic Torque Output Power ==
  note: Torque from Damper Windings
  note: Torque from Field Winding
  Id : Inport
  Iq : Inport  Port=2
  Eq1 : Inport  Port=3
  Ed1 : Inport  Port=4
  Phi_1d : Inport  Port=5
  Phi_2q : Inport  Port=6
  Gain : Gain  Gain=(Xd2 - Xls)/(Xd1 - Xls)
  Gain1 : Gain  Gain=(Xq2 - Xls)/(Xq1 - Xls)
  Gain2 : Gain  Gain=(Xd1 - Xd2)/(Xd1-Xls)
  Gain3 : Gain  Gain=(Xq1 - Xq2)/(Xq1-Xls)
  Gain4 : Gain  Gain=(Xq2 - Xd2)
  Product{,1..4} (5 alike) : Product  RndMeth=Zero
  Sum : Sum
  Sum1 : Sum  Inputs=+-+
  Sum2 : Sum
  TE : Outport
  wires:
  Sum2/1 -> TE/1
  Sum1/1 -> Sum2/2
  Sum/1 -> Sum2/1
  Gain1/1 -> Sum/2
  Gain/1 -> Sum/1
  Gain4/1 -> Sum1/3
  Gain2/1 -> Sum1/1
  Gain3/1 -> Sum1/2
  Product4/1 -> Gain4/1
  [Iq] -> Product4/2
  [Id] -> Product4/1
  Product3/1 -> Gain3/1
  [Phi_2q] -> Product3/2
  [Id] -> Product3/1
  Product2/1 -> Gain2/1
  [Phi_1d] -> Product2/2
  [Iq] -> Product2/1
  Product1/1 -> Gain1/1
  [Id] -> Product1/2
  [Ed1] -> Product1/1
  Product/1 -> Gain/1
  [Iq] -> Product/2
  [Eq1] -> Product/1
  Iq/1 -> [Iq]
  Phi_2q/1 -> [Phi_2q]
  Phi_1d/1 -> [Phi_1d]
  Ed1/1 -> [Ed1]
  Eq1/1 -> [Eq1]
  Id/1 -> [Id]

== system PowerFlowLib/Energy & Power Systems/Electrical/Machines/Synchronous Machine P.U. dq0/Generator Power Loss ==
  Ed : Inport
  Eq : Inport  Port=2
  Id : Inport  Port=3
  Iq : Inport  Port=4
  Te : Inport  Port=5
  w/ws : Inport  Port=6
  Bus Creator : BusCreator  Inputs=6
  Gain1 : Gain  Gain=SB
  Gain2 : Gain  Gain=SB
  Gain3 : Gain  Gain=SB
  Product : Product  RndMeth=Zero
  Product1 : Product  RndMeth=Zero
  Product2 : Product  RndMeth=Zero
  Sum1 : Sum  Inputs=-+
  Sum2 : Sum
  PE : Outport
  PM : Outport  Port=2
  PLOSS : Outport  Port=3
  m : Outport  Port=4
  wires:
  Gain3/1 -> PM/1
  Gain1/1 -> PE/1
  Gain2/1 -> PLOSS/1
  Bus Creator/1 -> m/1
  [nu] -> Bus Creator/6  "nu"
  [Te] -> Bus Creator/5  "Te"
  [Iq] -> Bus Creator/4  "Iq"
  [Eq] -> Bus Creator/3  "Vq"
  [Id] -> Bus Creator/2  "Id"
  [Ed] -> Bus Creator/1  "Vd"
  Sum1/1 -> Gain2/1
  Product2/1 -> Gain3/1, Sum1/2
  Sum2/1 -> Gain1/1, Sum1/1
  Product1/1 -> Sum2/2
  Product/1 -> Sum2/1
  [nu] -> Product2/2
  [Te] -> Product2/1
  [Iq] -> Product1/2
  [Eq] -> Product1/1
  [Id] -> Product/2
  [Ed] -> Product/1
  w/ws/1 -> [nu]
  Te/1 -> [Te]
  Iq/1 -> [Iq]
  Id/1 -> [Id]
  Eq/1 -> [Eq]
  Ed/1 -> [Ed]

== system PowerFlowLib/Energy & Power Systems/Electrical/Machines/Synchronous Machine P.U. dq0/Generator Power Loss1 ==
  Ploss : Inport
  Tamb : Inport  Port=2
  Gain1 : Gain  Gain=1/mc_gen
  Heat Trasnfer : Subsystem
  Integrator : Integrator  InitialConditionSource=external
  Sum : Sum  Inputs=|+-
  Ts : Outport
  Pdiss : Outport  Port=2
  wires:
  Gain1/1 -> Integrator/1
  Heat Trasnfer/1(Pdiss) -> Pdiss/1, Sum/2
  Ploss/1 -> Sum/1
  Sum/1 -> Gain1/1
  Integrator/1 -> Heat Trasnfer/2(Ts), Ts/1
  Tamb/1 -> Heat Trasnfer/1(Tamb), Integrator/2

== system PowerFlowLib/Energy & Power Systems/Electrical/Machines/Synchronous Machine P.U. dq0/Stator Voltage ==
  Id : Inport
  Iq : Inport  Port=2
  Eq1 : Inport  Port=3
  Ed1 : Inport  Port=4
  Phi_1d : Inport  Port=5
  Phi_2q : Inport  Port=6
  w/ws : Inport  Port=7
  Gain : Gain  Gain=(Xq2 - Xls)/(Xq1 - Xls)
  Gain1 : Gain  Gain=(Xq1 - Xq2)/(Xq1 - Xls)
  Gain2 : Gain  Gain=(Xq2 - Xd2)
  Gain3 : Gain  Gain=(Xd2 - Xls)/(Xd1 - Xls)
  Gain4 : Gain  Gain=(Xd1 - Xd2)/(Xd1 - Xls)
  Gain5 : Gain  Gain=Rs
  Gain6 : Gain  Gain=Xd2+XTL
  Gain7 : Gain  Gain=Rs+RTL
  Gain8 : Gain  Gain=Xd2+XTL
  Product{,1..3} (4 alike) : Product  RndMeth=Zero
  Sum : Sum
  Sum1 : Sum  Inputs=+-+
  Sum2 : Sum  Inputs=--+
  Sum3 : Sum  Inputs=-++
  Ed : Outport
  Eq : Outport  Port=2
  wires:
  Gain7/1 -> Sum2/2
  Product3/1 -> Sum2/1
  Sum2/1 -> Eq/1  "Vq"
  Sum3/1 -> Ed/1  "Vd"
  Product2/1 -> Sum3/3
  Gain2/1 -> Sum1/3
  Product1/1 -> Sum3/2
  Gain8/1 -> Product3/1
  Gain5/1 -> Sum3/1
  Gain6/1 -> Product2/2
  Id/1 -> Gain8/1, Gain5/1
  Product/1 -> Sum2/3
  w/ws/1 -> Product2/1, Product3/2, Product/2, Product1/2
  Sum1/1 -> Product1/1
  Sum/1 -> Product/1
  Gain1/1 -> Sum1/2
  Gain/1 -> Sum1/1
  Gain3/1 -> Sum/1
  Gain4/1 -> Sum/2
  Phi_1d/1 -> Gain4/1
  Eq1/1 -> Gain3/1
  Iq/1 -> Gain2/1, Gain7/1, Gain6/1
  Phi_2q/1 -> Gain1/1
  Ed1/1 -> Gain/1

== system PowerFlowLib/Energy & Power Systems/Electrical/Systems/Gen Bus w// APU switch/VOLTAGE FAULT DETECTION LOGIC ==
  note: This input determines the start of voltage monitoring
  In1 : Inport
  Constant1 : Constant  Value=LOWVLIMIT
  Constant2 : Constant  Value=UPVLIMIT
  Logical Operator : Logic  Operator=OR  AllPortsSameDT=off  OutDataTypeStr=boolean
  Logical Operator1 : Logic  Operator=NAND  AllPortsSameDT=off  OutDataTypeStr=boolean
  Relational Operator : RelationalOperator  Operator=<=  OutDataTypeStr=boolean  ZeroCross=off
  Relational Operator1 : RelationalOperator  OutDataTypeStr=boolean  ZeroCross=off
  Fault Signal (Acitve Low) : Outport
  wires:
  Logical Operator1/1 -> Fault Signal (Acitve Low)/1
  In1/1 -> Relational Operator1/1, Relational Operator/1
  [enable] -> Logical Operator1/2
  Logical Operator/1 -> Logical Operator1/1
  Relational Operator1/1 -> Logical Operator/2
  Relational Operator/1 -> Logical Operator/1
  Constant2/1 -> Relational Operator1/2
  Constant1/1 -> Relational Operator/2

== system PowerFlowLib/Energy & Power Systems/Electrical/Systems/Generation Unit Sync-Sync/Chopper (Averaged) ==
  vin : Inport
  q : Inport  Port=2
  Temperature : Inport  Port=3
  1/R : Gain  Gain=1/(R_fd_exc*VBFD_exc/IBFD_exc)/100/2*3/100  SaturateOnIntegerOverflow=on  OutDataTypeStr=Inherit: Same as input  ParamDataTypeStr=Inherit: Same as input
  Divide : Product  Inputs=*/
  Dot Product : DotProduct  InputSameDT=on  OutDataTypeStr=Inherit: Inherit via internal rule
  Dot Product1 : DotProduct  InputSameDT=on  OutDataTypeStr=Inherit: Inherit via internal rule
  Gain2 : Gain  Gain=1000*2/3
  Saturation : Saturate  UpperLimit=1  LowerLimit=0
  iout : Outport
  iin : Outport  Port=2
  wires:
  Dot Product1/1 -> iin/1
  Saturation/1 -> Dot Product1/2, Dot Product/2
  Dot Product/1 -> 1/R/1
  q/1 -> Saturation/1
  vin/1 -> Dot Product/1
  Gain2/1 -> Dot Product1/1, iout/1
  1/R/1 -> Divide/1
  Temperature/1 -> Divide/2
  Divide/1 -> Gain2/1
